simulink model "nodal"  (R2015a)
settings: Solver=ode45  StartTime=0.0  StopTime=10.0  RelTol=1e-3
libraries: fl_lib x9, nesl_utility x3
settings Model: Creator=ASUS  LastModifiedBy=ASUS

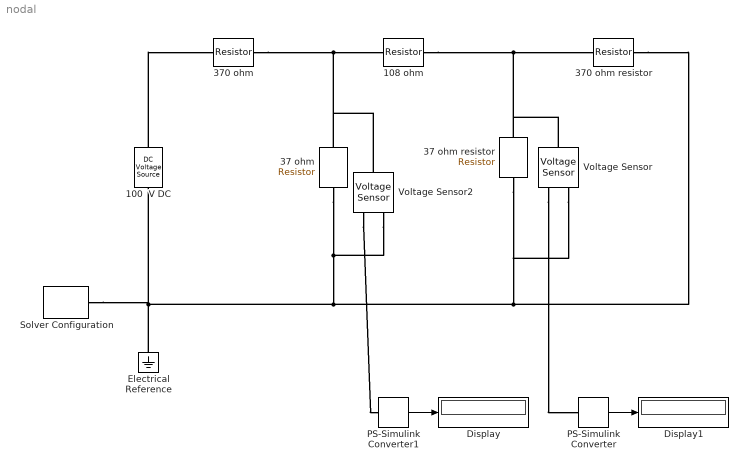
== system nodal ==
  " 108 ohm" : fl_lib/Electrical/Electrical Elements/Resistor  R=108 Ohm  i_specify=off  i_priority=High  i=0 A  v_specify=off  v_priority=High  v=0 V
  " 37 ohm resistor" : fl_lib/Electrical/Electrical Elements/Resistor  R=37 Ohm  i_specify=off  i_priority=High  i=0 A  v_specify=off  v_priority=High  v=0 V
  100  V DC : fl_lib/Electrical/Electrical Sources/DC Voltage Source  v0=100 V
  37 ohm : fl_lib/Electrical/Electrical Elements/Resistor  R=37 Ohm  i_specify=off  i_priority=High  i=0 A  v_specify=off  v_priority=High  v=0 V
  370 ohm : fl_lib/Electrical/Electrical Elements/Resistor  R=370 Ohm  i_specify=off  i_priority=High  i=0 A  v_specify=off  v_priority=High  v=0 V
  370 ohm resistor : fl_lib/Electrical/Electrical Elements/Resistor  R=370 Ohm  i_specify=off  i_priority=High  i=0 A  v_specify=off  v_priority=High  v=0 V
  Display : Display
  Display1 : Display
  Electrical Reference : fl_lib/Electrical/Electrical Elements/Electrical Reference
  PS-Simulink Converter : nesl_utility/PS-Simulink Converter  PhysicalDomain=network_engine_domain  SubClassName=ps_output  LeftPortType=input  RightPortType=output  PseudoPeriodic=off  Frequencies=[]  Unit=1  AffineConversion=off
  PS-Simulink Converter1 : nesl_utility/PS-Simulink Converter  PhysicalDomain=network_engine_domain  SubClassName=ps_output  LeftPortType=input  RightPortType=output  PseudoPeriodic=off  Frequencies=[]  Unit=1  AffineConversion=off
  Solver Configuration : nesl_utility/Solver Configuration  PhysicalDomain=network_engine_domain  SubClassName=solver  LeftPortType=input  RightPortType=generic  Accelerate=off  Tones=[]  Harmonics=[]  SimulateNoise=off  Profile=off  UseLocalSampling=off  EnableSwitchedLinearOptims=on  FrequencyDomain=off  UseCCode=off  RelTol=0.001  AbsTol=1e-06  MinStep=1e-09  ToWorkspace=off  RevertToSquareIcSolve=off  NumHomotopyIterations=100  DoDC=off  ResidualTolerance=1e-09  UseLocalSolver=off  LocalSolverChoice=NE_BACKWARD_EULER_ADVANCER  LocalSolverSampleTime=0.001  DoFixedCost=off  MaxNonlinIter=3  MaxModeIter=2  LinearAlgebra=Sparse  DelaysMemoryBudget=1024  AutomaticFiltering=on  FilteringTimeConstant=0.001
  Voltage Sensor : fl_lib/Electrical/Electrical Sensors/Voltage Sensor
  Voltage Sensor2 : fl_lib/Electrical/Electrical Sensors/Voltage Sensor
  wires:
  PS-Simulink Converter1/1 -> Display/1
  PS-Simulink Converter/1 -> Display1/1
  connections:
  100  V DC/LConn1 -- 370 ohm/LConn1
  370 ohm/RConn1 -- Voltage Sensor2/LConn1 -- 37 ohm/LConn1 -- " 108 ohm"/LConn1
  " 108 ohm"/RConn1 -- Voltage Sensor/LConn1 -- " 37 ohm resistor"/LConn1 -- 370 ohm resistor/LConn1
  37 ohm/RConn1 -- Voltage Sensor2/RConn2 -- Voltage Sensor/RConn2 -- " 37 ohm resistor"/RConn1 -- 370 ohm resistor/RConn1 -- Electrical Reference/LConn1 -- Solver Configuration/RConn1 -- 100  V DC/RConn1
  Voltage Sensor2/RConn1 -- PS-Simulink Converter1/LConn1
  Voltage Sensor/RConn1 -- PS-Simulink Converter/LConn1
